simulink model "quarterCar"  (R2023b)
settings: Solver=VariableStepAuto  StartTime=0.0  StopTime=15  RelTol=1e-3
libraries: SignalEditorBlockLib x1
settings Model: Creator=jackychen  LastModifiedBy=jackychen

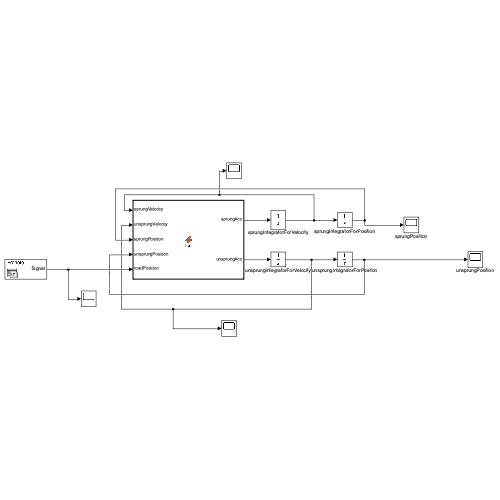
[thumbnail: Simulink's stored preview of the top-level diagram]
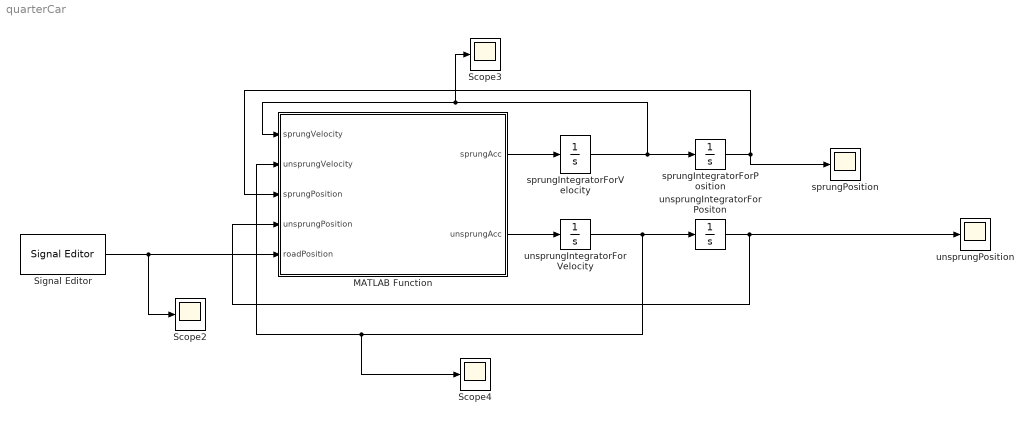
== system quarterCar ==
  MATLAB Function : MATLAB Function  TreatAsAtomicUnit=on
  Scope2 : Scope
  Scope3 : Scope
  Scope4 : Scope
  Signal Editor : SignalEditorBlockLib/Signal Editor  FileName=Test.mat  ActiveScenario=Pothole  ActiveSignal=Signal  IsBus=off  OutputBusObjectStr=Bus: BusObject  SampleTime=0  ZeroCross=off  OutputAfterFinalValue=Setting to zero  Unit=inherit  PreserveSignalName=on  ApplySigPropsToAllScenarios=on  ApplySigPropsToAllSignals=off
  sprungIntegratorForPosition : Integrator
  sprungIntegratorForVelocity : Integrator
  sprungPosition : Scope
  unsprungIntegratorForPositon : Integrator
  unsprungIntegratorForVelocity : Integrator
  unsprungPosition : Scope
  wires:
  MATLAB Function/1(sprungAcc) -> sprungIntegratorForVelocity/1
  sprungIntegratorForVelocity/1 -> Scope3/1, MATLAB Function/1(sprungVelocity), sprungIntegratorForPosition/1
  MATLAB Function/2(unsprungAcc) -> unsprungIntegratorForVelocity/1
  unsprungIntegratorForVelocity/1 -> Scope4/1, MATLAB Function/2(unsprungVelocity), unsprungIntegratorForPositon/1
  unsprungIntegratorForPositon/1 -> unsprungPosition/1, MATLAB Function/4(unsprungPosition)
  Signal Editor/1 -> MATLAB Function/5(roadPosition), Scope2/1
  sprungIntegratorForPosition/1 -> sprungPosition/1, MATLAB Function/3(sprungPosition)

== matlab function quarterCar/MATLAB Function ==
  data: sprungVelocity input; unsprungVelocity input; sprungPosition input; unsprungPosition input; sprungAcc output; unsprungAcc output; roadPosition input
function [sprungAcc, unsprungAcc]= fcn(sprungVelocity, unsprungVelocity, sprungPosition, unsprungPosition, roadPosition)
grav = 9.81;
sprungMass = 50;
sprungDamperConst = 500;
sprungSpringConst = 50000;
tireSpringConst = 127000;
unsprungMass = 10;

% Delta x for spring force
sprungDeltax = sprungPosition - unsprungPosition;
unsprungDeltax = unsprungPosition - roadPosition;

%Spring Force
sprungSpringForce = -(sprungSpringConst * sprungDeltax);
tireSpringForce = -(tireSpringConst * unsprungDeltax);

%netVelocity for damper
netVelocity = sprungVelocity - unsprungVelocity;

% Calculations here

sprungAcc = ((-sprungDamperConst * netVelocity) + (sprungSpringForce) - (sprungMass * grav)) / (sprungMass);

unsprungAcc =  ((tireSpringForce) - (sprungSpringForce) + (sprungDamperConst * netVelocity) - (unsprungMass*grav)) / (unsprungMass);
